simulink model "sequence_generation"  (Simulink 6.6)
settings: Solver=VariableStepDiscrete  StartTime=0.0  StopTime=512/28e6  RelTol=1e-3
StopFcn:
  | figure(1)
  | plot(I_channel,Q_channel,'ko','MarkerFaceColor','b');
  | xlabel('I channel');
  | ylabel('Q_channel');
  | title('64 QAM Constellation');
settings Model: Creator=lcrockett  LastModifiedBy=lcrockett
settings OptimizationCC: InlineParams=on  InlineInvariantSignals=on
settings DebuggingCC: SignalResolutionControl=TryResolveAllWithWarning  MultiTaskDSMMsg=warning  MultiTaskCondExecSysMsg=none  StrictBusMsg=None
settings RTWCC: IncludeERTFirstTime=on

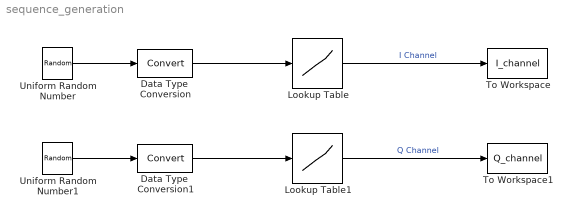
== system sequence_generation ==
  Data Type  Conversion : DataTypeConversion  OutDataTypeMode=Specify via dialog  OutDataType=uint(3)  RndMeth=Nearest  SaturateOnIntegerOverflow=on
  Data Type  Conversion1 : DataTypeConversion  OutDataTypeMode=Specify via dialog  OutDataType=uint(3)  RndMeth=Nearest  SaturateOnIntegerOverflow=on
  Lookup Table : Lookup  InputValues=[0 1 2 3 4 5 6 7]  OutputValues=[127 90.71428571 54.42857143 18.14285714 -18.14285714 -54.42857143 -90.71428571 -127]  OutDataTypeMode=Specify via dialog  OutDataType=float('double')
  Lookup Table1 : Lookup  InputValues=[0 1 2 3 4 5 6 7]  OutputValues=[127 90.71428571 54.42857143 18.14285714 -18.14285714 -54.42857143 -90.71428571 -127]  OutDataTypeMode=Specify via dialog  OutDataType=float('double')
  To Workspace : ToWorkspace  VariableName=I_channel  SampleTime=-1  SaveFormat=Array
  To Workspace1 : ToWorkspace  VariableName=Q_channel  SampleTime=-1  SaveFormat=Array
  Uniform Random Number : UniformRandomNumber  Minimum=0  Maximum=7  SampleTime=1/28e6
  Uniform Random Number1 : UniformRandomNumber  Minimum=0  Maximum=7  Seed=1  SampleTime=1/28e6
  wires:
  Uniform Random Number/1 -> Data Type  Conversion/1
  Data Type  Conversion1/1 -> Lookup Table1/1
  Uniform Random Number1/1 -> Data Type  Conversion1/1
  Lookup Table/1 -> To Workspace/1  "I Channel"
  Lookup Table1/1 -> To Workspace1/1  "Q Channel"
  Data Type  Conversion/1 -> Lookup Table/1
